simulink model "Fig275"  (R2014b)
settings: Solver=ode3  StartTime=0.0  StopTime=1  FixedStep=2e-5  RelTol=1e-5
libraries: commutil2 x1, dsparch4 x1, commrandsrc2 x1
settings Model: Creator=Dennis Silage  LastModifiedBy=Silage
settings DataIOCC: SignalLoggingSaveFormat=ModelDataLogs
settings OptimizationCC: ExpressionDepthLimit=2147483647  InitFltsAndDblsToZero=on
settings DebuggingCC: UnderspecifiedInitializationDetection=Classic  MergeDetectMultiDrivingBlocksExec=none  SolverPrmCheckMsg=none  FcnCallInpInsideContextMsg=UseLocalSettings  StateNameClashWarn=warning
settings GRTTargetCC: CombineOutputUpdateFcns=off  GRTInterface=on

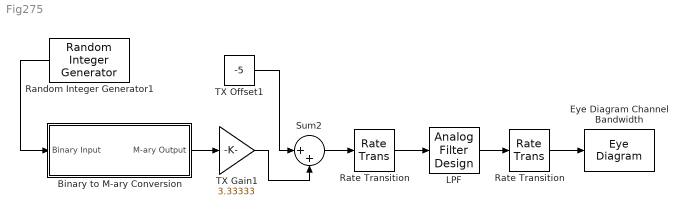
== system Fig275 ==
  Binary to M-ary Conversion : Subsystem
  Eye Diagram Channel Bandwidth : EyeDiagram  Tag=EyeDiagram
  LPF : dsparch4/Analog Filter Design  method=Chebyshev I  filttype=Lowpass  N=9  Wlo=2*pi*1200  Whi=80  Rp=0.1  Rs=40
  Random Integer Generator1 : commrandsrc2/Random Integer Generator  mul=2  seed=randseed  Ts=1e-3  frameBased=off  sampPerFrame=1  orient=off  outDataType=double
  Rate Transition : RateTransition  OutPortSampleTime=2e-5
  "Rate Transition " : RateTransition  OutPortSampleTime=2e-5
  Sum2 : Sum  Inputs=|++
  TX Gain1 : Gain  Gain=3.33333
  TX Offset1 : Constant  Value=-5
  wires:
  LPF/1 -> "Rate Transition "/1
  Random Integer Generator1/1 -> Binary to M-ary Conversion/1(Binary Input)
  TX Gain1/1 -> Sum2/2
  TX Offset1/1 -> Sum2/1
  Binary to M-ary Conversion/1("M-ary Output ") -> TX Gain1/1
  Rate Transition/1 -> LPF/1
  Sum2/1 -> Rate Transition/1
  "Rate Transition "/1 -> Eye Diagram Channel Bandwidth/1

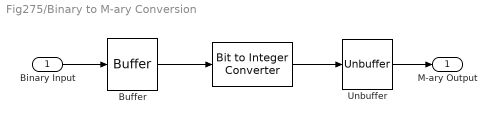
== system Fig275/Binary to M-ary Conversion ==
  Binary Input : Inport
  " " : commutil2/Bit to Integer Converter  nbits=2  bitOrder=MSB first  signedOutputValues=Unsigned  outDtype=Inherit via internal rule  outDtypeSigned=Inherit via internal rule
  Buffer : Buffer  N=2  TreatMby1Signals=One channel
  Unbuffer : Unbuffer  SampleBasedProcessing=Same as frame based
  "M-ary Output " : Outport
  wires:
  Binary Input/1 -> Buffer/1
  Buffer/1 -> " "/1
  " "/1 -> Unbuffer/1
  Unbuffer/1 -> "M-ary Output "/1
